simulink model "pt2_blockdiagram"  (R2019a)
settings: Solver=ode4  StartTime=0.0  StopTime=20e-3  FixedStep=0.3e-3  RelTol=1e-3  EnableMultiTasking=on
InitFcn:
  | pt2_data;
values from neighbouring files (symbols this model uses):
  P_D = 0.3    [pt2_data.m]
  P_k = 1    [pt2_data.m]
  P_T = 1e-3    (= 0.001)    [pt2_data.m]
  P_v0 = 0    [pt2_data.m]
  P_x0 = 0    [pt2_data.m]
settings Model: Creator=traenkle  LastModifiedBy=ftraenkle
settings DataIOCC: LimitDataPoints=on  SaveFormat=Array  InspectSignalLogs=on  ReturnWorkspaceOutputs=off
settings OptimizationCC: LifeSpan=inf
settings DebuggingCC: UnderspecifiedInitializationDetection=Classic  MergeDetectMultiDrivingBlocksExec=none  SolverPrmCheckMsg=warning  MultiTaskDSMMsg=warning  MultiTaskCondExecSysMsg=none  AllowSymbolicDim=off  StateNameClashWarn=warning  SFUnexpectedBacktrackingDiag=warning  SFNoUnconditionalDefaultTransitionDiag=warning  SFExecutionAtInitializationDiag=none  ArithmeticOperatorsInVariantConditions=warning
settings HardwareCC: ProdBitPerPointer=32  ProdBitPerSizeT=32  ProdBitPerPtrDiffT=32  ProdLargestAtomicFloat=None  ProdIntDivRoundTo=Undefined  ProdEndianess=Unspecified  ProdWordSize=32  ProdHWDeviceType=32-bit Generic
settings ModelReferenceCC: PropagateSignalLabelsOutOfModel=off
settings SFSimCC: SimUseLocalCustomCode=off
settings RTWCC: RTWUseLocalCustomCode=off
settings CodeAppCC: StateflowObjectComments=on
settings GRTTargetCC: TargetLangStandard=C89/C90 (ANSI)
settings ConfigComp: CovMetricSettings=dw  CovSaveCumulativeToWorkspaceVar=on  CovSaveSingleToWorkspaceVar=on  CovExternalEMLEnable=off

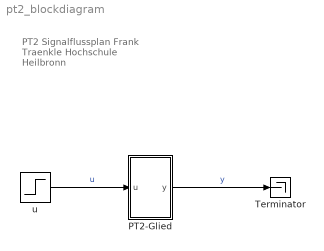
== system pt2_blockdiagram ==
  note: PT2 Signalflussplan
      | Frank Traenkle
      | Hochschule Heilbronn
  PT2-Glied : Subsystem
  Terminator : Terminator
  u : Step  Time=0  SampleTime=0
  wires:
  u/1 -> PT2-Glied/1(u)  "u"
  PT2-Glied/1(y) -> Terminator/1  "y"

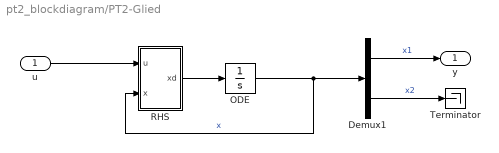
== system pt2_blockdiagram/PT2-Glied ==
  u : Inport
  Demux1 : Demux  Outputs=2
  ODE : Integrator  InitialCondition=[ P_x0 ; P_v0 ]
  RHS : Subsystem
  Terminator : Terminator
  y : Outport  VectorParamsAs1DForOutWhenUnconnected=off
  wires:
  ODE/1 -> RHS/2(x), Demux1/1  "x"
  Demux1/1 -> y/1  "x1"
  Demux1/2 -> Terminator/1  "x2"
  RHS/1(xd) -> ODE/1
  u/1 -> RHS/1(u)

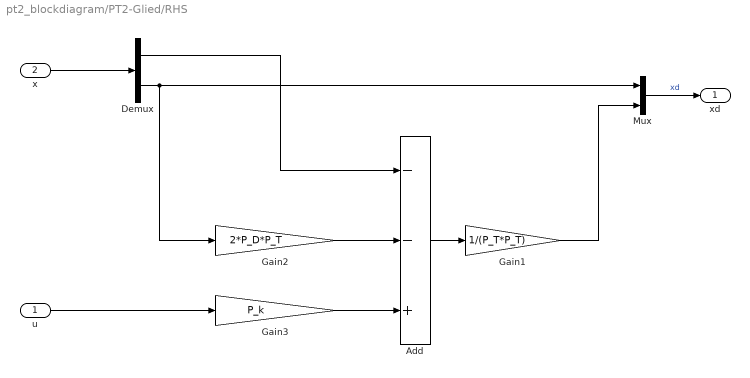
== system pt2_blockdiagram/PT2-Glied/RHS ==
  u : Inport
  x : Inport  Port=2
  Add : Sum  Inputs=--+
  Demux : Demux  Outputs=2
  Gain1 : Gain  Gain=1/(P_T*P_T)
  Gain2 : Gain  Gain=2*P_D*P_T
  Gain3 : Gain  Gain=P_k
  Mux : Mux  Inputs=2
  xd : Outport  VectorParamsAs1DForOutWhenUnconnected=off
  wires:
  Mux/1 -> xd/1  "xd"
  Demux/2 -> Gain2/1, Mux/1
  x/1 -> Demux/1
  u/1 -> Gain3/1
  Gain3/1 -> Add/3
  Gain2/1 -> Add/2
  Demux/1 -> Add/1
  Add/1 -> Gain1/1
  Gain1/1 -> Mux/2
